simulink model "model_simulink"  (R2019a)
settings: Solver=VariableStepAuto  StartTime=0.0  StopTime=Tsim  RelTol=1e-3
values from neighbouring files (symbols this model uses):
  Fsin = 3    [script_matlab.m]
  Te = 1/Fe    (= 3.125e-06)    [Simulation_projet.m]    (also in script_matlab.m = 0.03125)
settings Model: Creator=gonzalve  LastModifiedBy=gonzalve

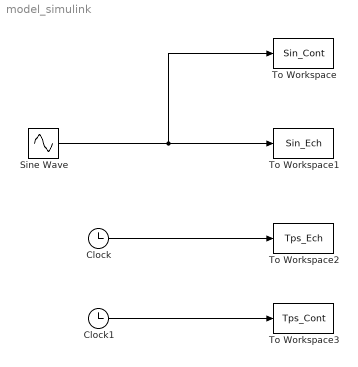
== system model_simulink ==
  Clock : Clock
  Clock1 : Clock
  Sine Wave : Sin  Frequency=Fsin  SampleTime=0
  To Workspace : ToWorkspace  VariableName=Sin_Cont  SampleTime=Te/100
      settings: Save2DSignal=2-D array (concatenate along first dimension)
  To Workspace1 : ToWorkspace  VariableName=Sin_Ech  SampleTime=Te
      settings: Save2DSignal=2-D array (concatenate along first dimension)
  To Workspace2 : ToWorkspace  VariableName=Tps_Ech  SampleTime=Te
      settings: Save2DSignal=2-D array (concatenate along first dimension)
  To Workspace3 : ToWorkspace  VariableName=Tps_Cont  SampleTime=Te/100
      settings: Save2DSignal=2-D array (concatenate along first dimension)
  wires:
  Clock/1 -> To Workspace2/1
  Clock1/1 -> To Workspace3/1
  Sine Wave/1 -> To Workspace/1, To Workspace1/1
